simulink library "DYN_TIME"  (Simulink 10.1)
settings: Solver=VariableStepAuto  StartTime=0.0  StopTime=10.0  RelTol=1e-3
libraries: LIB_TIME x1
settings Model: Creator=Mahal  LastModifiedBy=m_mam

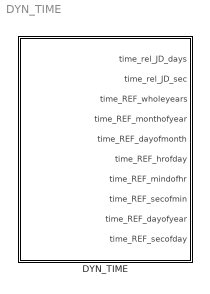
== system DYN_TIME ==
  DYN_TIME : Subsystem

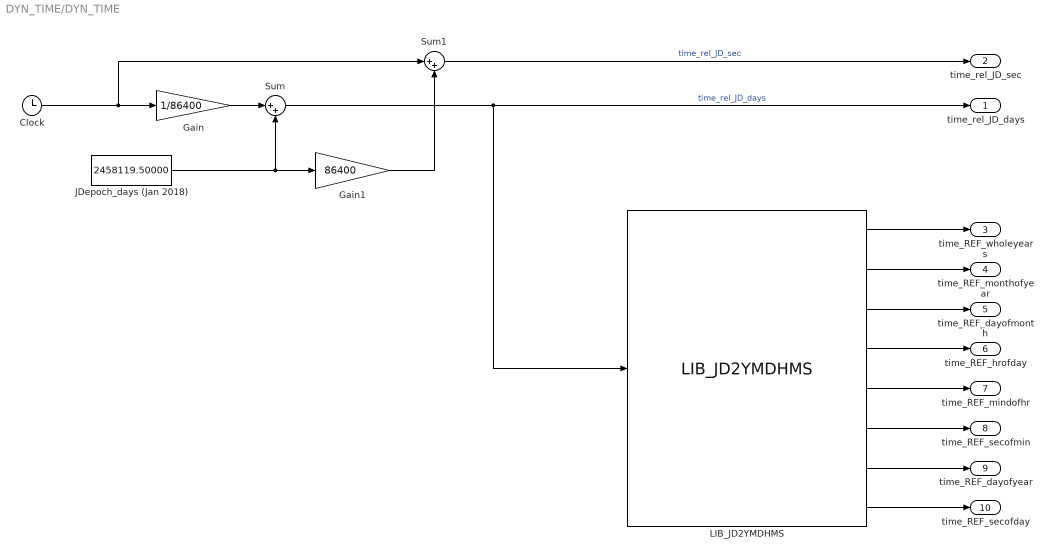
== system DYN_TIME/DYN_TIME ==
  Clock : Clock
  Gain : Gain  Gain=1/86400
  Gain1 : Gain  Gain=86400
  JDepoch_days (Jan 2018) : Constant  Value=2458119.50000
  LIB_JD2YMDHMS : LIB_TIME/LIB_JD2YMDHMS  SystemSampleTime=-1  Latency=0  AutoFrameSizeCalculation=off
  Sum : Sum  Inputs=|++
  Sum1 : Sum  Inputs=|++
  time_rel_JD_days : Outport  VectorParamsAs1DForOutWhenUnconnected=off
  time_rel_JD_sec : Outport  Port=2  VectorParamsAs1DForOutWhenUnconnected=off
  time_REF_wholeyears : Outport  Port=3  VectorParamsAs1DForOutWhenUnconnected=off
  time_REF_monthofyear : Outport  Port=4  VectorParamsAs1DForOutWhenUnconnected=off
  time_REF_dayofmonth : Outport  Port=5  VectorParamsAs1DForOutWhenUnconnected=off
  time_REF_hrofday : Outport  Port=6  VectorParamsAs1DForOutWhenUnconnected=off
  time_REF_mindofhr : Outport  Port=7  VectorParamsAs1DForOutWhenUnconnected=off
  time_REF_secofmin : Outport  Port=8  VectorParamsAs1DForOutWhenUnconnected=off
  time_REF_dayofyear : Outport  Port=9  VectorParamsAs1DForOutWhenUnconnected=off
  time_REF_secofday : Outport  Port=10  VectorParamsAs1DForOutWhenUnconnected=off
  wires:
  LIB_JD2YMDHMS/2 -> time_REF_monthofyear/1
  LIB_JD2YMDHMS/1 -> time_REF_wholeyears/1
  LIB_JD2YMDHMS/3 -> time_REF_dayofmonth/1
  Gain1/1 -> Sum1/2
  LIB_JD2YMDHMS/4 -> time_REF_hrofday/1
  LIB_JD2YMDHMS/7 -> time_REF_dayofyear/1
  Sum1/1 -> time_rel_JD_sec/1  "time_rel_JD_sec"
  LIB_JD2YMDHMS/8 -> time_REF_secofday/1
  Sum/1 -> LIB_JD2YMDHMS/1, time_rel_JD_days/1  "time_rel_JD_days"
  LIB_JD2YMDHMS/6 -> time_REF_secofmin/1
  Gain/1 -> Sum/1
  LIB_JD2YMDHMS/5 -> time_REF_mindofhr/1
  JDepoch_days (Jan 2018)/1 -> Gain1/1, Sum/2
  Clock/1 -> Sum1/1, Gain/1
